simulink model "model"  (R2020b)
settings: Solver=VariableStepAuto  StartTime=0.0  StopTime=10.0  RelTol=1e-3
values from neighbouring files (symbols this model uses):
  B = 1e-6    (= 1e-06)    [intialize_input.m]
  J = 15.17e-6    (= 1.517e-05)    [intialize_input.m]
  Ke = 56.23e-6    (= 5.623e-05)    [intialize_input.m]
  L = 5.05e-3    (= 0.00505)    [intialize_input.m]
  P = 4    [intialize_input.m]
  R = 4.98    [intialize_input.m]
  Tm = 0.1    [intialize_input.m]
  Va = 30    [intialize_input.m]
  Vb = 0    [intialize_input.m]
  Vc = 0    [intialize_input.m]
settings Model: Creator=Vrunda M Balgi  LastModifiedBy=Vrunda M Balgi
settings DataIOCC: ExternalInput=[t, Va,Vb,Vc]  LoadExternalInput=on  ReturnWorkspaceOutputs=off

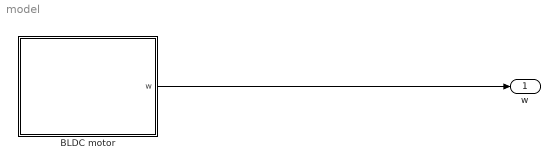
== system model ==
  BLDC motor : Subsystem
  w : Outport
  wires:
  BLDC motor/1(w) -> w/1

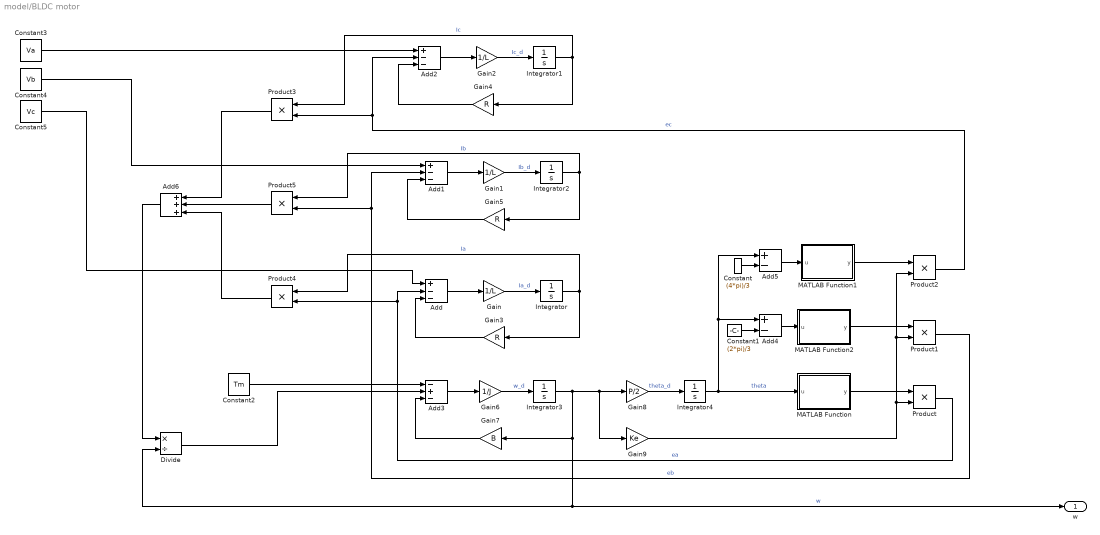
== system model/BLDC motor ==
  Add : Sum  Inputs=+--
  Add1 : Sum  Inputs=+--
  Add2 : Sum  Inputs=+--
  Add3 : Sum  Inputs=-+-
  Add4 : Sum  Inputs=+-
  Add5 : Sum  Inputs=+-
  Add6 : Sum  Inputs=+++
  Constant : Constant  Value=(4*pi)/3
  Constant1 : Constant  Value=(2*pi)/3
  Constant2 : Constant  Value=Tm
  Constant3 : Constant  Value=Va
  Constant4 : Constant  Value=Vb
  Constant5 : Constant  Value=Vc
  Divide : Product  Inputs=*/
  Gain : Gain  Gain=1/L
  Gain1 : Gain  Gain=1/L
  Gain2 : Gain  Gain=1/L
  Gain3 : Gain  Gain=R
  Gain4 : Gain  Gain=R
  Gain5 : Gain  Gain=R
  Gain6 : Gain  Gain=1/J
  Gain7 : Gain  Gain=B
  Gain8 : Gain  Gain=P/2
  Gain9 : Gain  Gain=Ke
  Integrator{,1..4} (5 alike) : Integrator
  MATLAB Function : MATLAB Function  TreatAsAtomicUnit=on
  MATLAB Function1 : MATLAB Function  TreatAsAtomicUnit=on
  MATLAB Function2 : MATLAB Function  TreatAsAtomicUnit=on
  Product{,1..5} (6 alike) : Product
  w : Outport
  wires:
  Gain9/1 -> Product2/2, Product1/2, Product/2
  Gain1/1 -> Integrator2/1  "Ib_d"
  Integrator/1 -> Gain3/1, Product4/1  "Ia"
  Integrator2/1 -> Gain5/1, Product5/1  "Ib"
  Integrator3/1 -> Gain8/1, Gain9/1, Gain7/1, w/1, Divide/2  "w"
  Add5/1 -> MATLAB Function1/1(u)
  Gain/1 -> Integrator/1  "Ia_d"
  MATLAB Function1/1(y) -> Product2/1
  Add2/1 -> Gain2/1
  Product2/1 -> Add2/2, Product3/2  "ec"
  Constant5/1 -> Add/1
  Gain3/1 -> Add/3
  Product5/1 -> Add6/2
  Integrator1/1 -> Gain4/1, Product3/1  "Ic"
  Gain5/1 -> Add1/3
  Integrator4/1 -> MATLAB Function/1(u), Add5/1, Add4/1  "theta"
  Add/1 -> Gain/1
  Add3/1 -> Gain6/1
  Gain2/1 -> Integrator1/1  "Ic_d"
  Add6/1 -> Divide/1
  Constant1/1 -> Add4/2
  Constant/1 -> Add5/2
  MATLAB Function2/1(y) -> Product1/1
  Gain7/1 -> Add3/3
  Product4/1 -> Add6/3
  Gain6/1 -> Integrator3/1  "w_d"
  Constant3/1 -> Add2/1
  Gain8/1 -> Integrator4/1  "theta_d"
  MATLAB Function/1(y) -> Product/1
  Product/1 -> Product4/2, Add/2  "ea"
  Product1/1 -> Product5/2, Add1/2  "eb"
  Divide/1 -> Add3/2
  Gain4/1 -> Add2/3
  Constant4/1 -> Add1/1
  Add1/1 -> Gain1/1
  Product3/1 -> Add6/1
  Constant2/1 -> Add3/1
  Add4/1 -> MATLAB Function2/1(u)

== matlab function model/BLDC motor/MATLAB Function ==
  data: u input; y output
function y = fcn(u)

if (u>=0 && u<((2*pi)/3))
    y = 1;
elseif(u>=((2*pi)/3) && u<pi)
    y = 1-(6/pi*(u-((2*pi)/3)));
elseif(u>=pi && u<((5*pi)/3))
    y = -1;
else
    y = -1+(6/pi*(u-((5*pi)/3)));
end
end

== matlab function model/BLDC motor/MATLAB Function2 ==
  data: u input; y output
function y = fcn(u)

if (u>=0 && u<((2*pi)/3))
    y = 1;
elseif(u>=((2*pi)/3) && u<pi)
    y = 1-(6/pi*(u-((2*pi)/3)));
elseif(u>=pi && u<((5*pi)/3))
    y = -1;
else
    y = -1+(6/pi*(u-((5*pi)/3)));
end
end

== matlab function model/BLDC motor/MATLAB Function1 ==
  data: u input; y output
function y = fcn(u)

if (u>=0 && u<((2*pi)/3))
    y = 1;
elseif(u>=((2*pi)/3) && u<pi)
    y = 1-(6/pi*(u-((2*pi)/3)));
elseif(u>=pi && u<((5*pi)/3))
    y = -1;
else
    y = -1+(6/pi*(u-((5*pi)/3)));
end
end
